simulink model "pacemaker_project_hw_system"  (R2021a)
settings: Solver=FixedStepDiscrete  StartTime=0.0  StopTime=50  FixedStep=1e-3  RelTol=1e-3  EnableMultiTasking=on
model workspace (MAT data in the model file):
  DefaultDataStore = 60
undefined symbols (not defined in the file): A3, A4, D0, D1, D10, D11, D12, D13, D2, D3, D4, D5, D6, D7, D8, D9, PTA0, PTA1, PTA2, PTB11, PTB23, PTB9, PTC11, PTC16, PTC17, PTC2, PTC3, PTC4, PTD0, PTD1, PTD2, PTD3
libraries: frdmk64flib x22, etargetslib x8, dspstat3 x1
settings Model: ExtModeTrigDuration=5  Creator=ali2h  LastModifiedBy=Razan
settings OptimizationCC: EnhancedBackFolding=on  PassReuseOutputArgsAs=Individual arguments  ZeroExternalMemoryAtStartup=off  ZeroInternalMemoryAtStartup=off  MaxStackSize=64  OptimizeBlockOrder=speed  DifferentSizesBufferReuse=on  OptimizationCustomize=off  EfficientTunableParamExpr=on
settings DebuggingCC: ParameterTunabilityLossMsg=error
settings HardwareCC: ProdBitPerPointer=32  ProdBitPerSizeT=32  ProdBitPerPtrDiffT=32  ProdLargestAtomicInteger=Long  ProdLargestAtomicFloat=Double  ProdWordSize=32  ProdHWDeviceType=ARM Compatible->ARM Cortex
settings SFSimCC: MATLABDynamicMemAlloc=off
settings RTWCC: SystemTargetFile=ert.tlc  HardwareBoard=NXP FRDM-K64F  TLCOptions="-aInlineSetEventsForThisBaseRateFcn=TLC_FALSE -aSuppressMultiTaskScheduler=TLC_FALSE  -aRateBasedStepFcn=0"  TemplateMakefile=ert_default_tmf  Toolchain=GNU Tools for ARM Embedded Processors
settings CodeAppCC: ForceParamTrailComments=on  IgnoreCustomStorageClasses=off  OperatorAnnotations=on  SimulinkDataObjDesc=on  SFDataObjDesc=on  InsertBlockDesc=on
settings ERTTargetCC: ExtModeTransport=4  ExtModeMexFile=sendToCommService

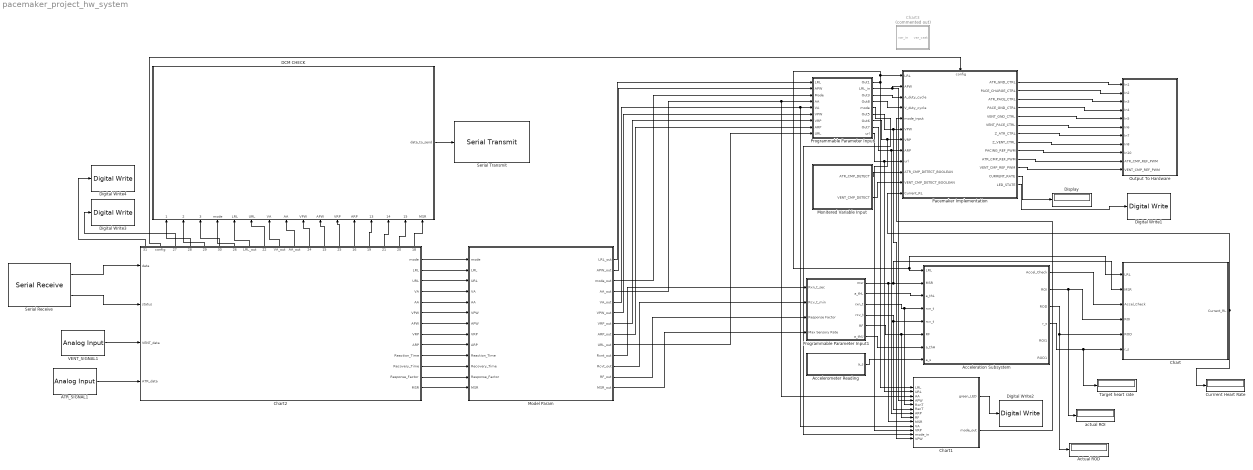
== system pacemaker_project_hw_system ==
  ATR_SIGNAL1 : frdmk64flib/Analog Input  Whichpin=PTB11 (A3)  SampleTime=-1
  Acceleration Subsystem : Subsystem
  Accelerometer Reading : Subsystem
  Actual ROD : Display
  Chart : Stateflow chart  TreatAsAtomicUnit=on
      settings: PortSchema="{\"entries\":[{\"content\":{\"sides\":[{\"content\":{\"connectorIds\":[\"In5\",\"In2\",\"In1\",\"In3\",\"In4\",\"In6\"]},\"type\":\"ConnectorPlacement.EquallySpacedRectSide\",\"uuid\":\"e2faaf11-533e-4519-93e0-9386f0696ab0\"},{\"content\":{\"connectorIds\":[\"Out1\"],\"side\":\"RIGHT\"},\"type\":\"ConnectorPlacement.EquallySpacedRectSide\",\"uuid\":\"3d822896-3a5e-473f-9176-095876908580\"},{\"content\":{\"connectorIds\":[],\"side\":\"TOP\"},\"type\":\"ConnectorPlacement.EquallySpacedRectSide\",\"uuid\":\"9e71e4b9-0a05-47a2-8aca-96ebbea26fb4\"}]},\"type\":\"ConnectorPlacement.EquallySpacedConnector\",\"uuid\":\"95b0b788-f876-4603-914d-e98930842ebd\"}],\"packageUris\":[\"http://schema.mathworks.com/mf0/Connector/R2020b\"],\"version\":\"1.0\"}"
  Chart1 : Stateflow chart  TreatAsAtomicUnit=on
      settings: PortSchema="{\"entries\":[{\"content\":{\"sides\":[{\"content\":{\"connectorIds\":[\"In2\",\"In4\",\"In1\",\"In5\",\"In7\",\"In6\",\"In8\",\"In10\",\"In9\",\"In11\",\"In13\",\"In3\",\"In12\"]},\"type\":\"ConnectorPlacement.EquallySpacedRectSide\",\"uuid\":\"456a7d9e-f2dc-4248-8632-54977d3d0e8d\"},{\"content\":{\"connectorIds\":[\"Out1\",\"Out2\"],\"side\":\"RIGHT\"},\"type\":\"ConnectorPlacement.EquallySpacedRectSide\",\"uuid\":\"93618940-8d2c-4873-bbdd-898375b2771e\"},{\"content\":{\"connectorIds\":[],\"side\":\"TOP\"},\"type\":\"ConnectorPlacement.EquallySpacedRectSide\",\"uuid\":\"193f6807-1d54-4c84-841f-0b1b2c52bae8\"}]},\"type\":\"ConnectorPlacement.EquallySpacedConnector\",\"uuid\":\"4b66c94b-72ab-490e-aaca-3b2f913491ef\"}],\"packageUris\":[\"http://schema.mathworks.com/mf0/Connector/R2020b\"],\"version\":\"1.0\"}"
  Chart2 : Stateflow chart  TreatAsAtomicUnit=on
      settings: PortSchema="{\"entries\":[{\"content\":{\"sides\":[{\"content\":{\"connectorIds\":[\"In1\",\"In2\",\"In3\",\"In4\"]},\"type\":\"ConnectorPlacement.EquallySpacedRectSide\",\"uuid\":\"e0d71676-4635-4cc5-940f-d91659ea50ca\"},{\"content\":{\"connectorIds\":[\"Out2\",\"Out1\",\"Out3\",\"Out4\",\"Out5\",\"Out6\",\"Out7\",\"Out13\",\"Out8\",\"Out9\",\"Out10\",\"Out11\",\"Out12\"],\"side\":\"RIGHT\"},\"type\":\"ConnectorPlacement.EquallySpacedRectSide\",\"uuid\":\"0805dafd-7d20-457a-bd79-7666b5721266\"},{\"content\":{\"connectorIds\":[\"Out31\",\"Out32\",\"Out27\",\"Out28\",\"Out29\",\"Out30\",\"Out26\",\"Out17\",\"Out22\",\"Out23\",\"Out14\",\"Out24\",\"Out15\",\"Out25\",\"Out16\",\"Out19\",\"Out21\",\"Out20\",\"Out18\"],\"side\":\"TOP\"},\"type\":\"ConnectorPlacement.EquallySpacedRectSide\",\"uuid\":\"7dce37fb-9cbe-4aeb-8643-08c0d0009600\"},{\"content\":{\"connectorIds\":[],\"side\":\"BOTTOM\"},\"type\":\"ConnectorPlacement.EquallySpacedRectSide\",\"uuid\":\"8cb6d6e2-e19d-4465-a9e0-7af84bc91401\"}]},\"type\":\"ConnectorPlacement.EquallySpacedConnector\",\"uuid\":\"ce183338-3f92-497d-b3e5-2333b87263be\"}],\"packageUris\":[\"http://schema.mathworks.com/mf0/Connector/R2020b\"],\"version\":\"1.0\"}"
  Chart3 : Stateflow chart  Commented=on  TreatAsAtomicUnit=on
  Currrent Heart Rate : Display
  DCM CHECK : Subsystem
      settings: PortSchema="{\"entries\":[{\"content\":{\"sides\":[{\"content\":{\"connectorIds\":[]},\"type\":\"ConnectorPlacement.EquallySpacedRectSide\",\"uuid\":\"5070fca3-03db-4702-bf74-10cd169506b7\"},{\"content\":{\"connectorIds\":[\"Out1\"],\"side\":\"RIGHT\"},\"type\":\"ConnectorPlacement.EquallySpacedRectSide\",\"uuid\":\"a99172cf-9b5d-4dae-9e4a-5601bc613afa\"},{\"content\":{\"connectorIds\":[],\"side\":\"TOP\"},\"type\":\"ConnectorPlacement.EquallySpacedRectSide\",\"uuid\":\"54f3c445-ca02-417c-9800-ac4eb04fe443\"},{\"content\":{\"connectorIds\":[\"In1\",\"In2\",\"In3\",\"In4\",\"In5\",\"In6\",\"In7\",\"In8\",\"In9\",\"In10\",\"In11\",\"In12\",\"In13\",\"In14\",\"In15\",\"In16\"],\"side\":\"BOTTOM\"},\"type\":\"ConnectorPlacement.EquallySpacedRectSide\",\"uuid\":\"fd0aef12-eb6d-4507-9c8c-5c9fc9d3837d\"}]},\"type\":\"ConnectorPlacement.EquallySpacedConnector\",\"uuid\":\"2a8d6b9e-4cb8-4645-8e28-a1ce966e9c6c\"}],\"packageUris\":[\"http://schema.mathworks.com/mf0/Connector/R2020b\"],\"version\":\"1.0\"}"
  Digital Write1 : frdmk64flib/Digital Write  Whichpin=RED_LED
  Digital Write2 : frdmk64flib/Digital Write  Whichpin=GREEN_LED
  Digital Write3 : frdmk64flib/Digital Write  Whichpin=BLUE_LED
  Digital Write4 : frdmk64flib/Digital Write  Whichpin=PTD1 (D13)
  Display : Display
  Model Param : Subsystem
  Monitered Variable Input : Subsystem
  Output To Hardware : Subsystem
  Pacemaker Implementation : Stateflow chart
      settings: PortSchema="{\"entries\":[{\"content\":{\"sides\":[{\"content\":{\"connectorIds\":[\"In2\",\"In3\",\"In4\",\"In5\",\"In6\",\"In7\",\"In8\",\"In9\",\"In13\",\"In10\",\"In11\",\"In12\"]},\"type\":\"ConnectorPlacement.EquallySpacedRectSide\",\"uuid\":\"2c436aae-0e07-4bda-8b45-2f1ae7c6679d\"},{\"content\":{\"connectorIds\":[\"Out1\",\"Out2\",\"Out3\",\"Out4\",\"Out5\",\"Out6\",\"Out7\",\"Out8\",\"Out9\",\"Out10\",\"Out11\",\"Out12\",\"Out13\"],\"side\":\"RIGHT\"},\"type\":\"ConnectorPlacement.EquallySpacedRectSide\",\"uuid\":\"f66ba986-5db0-4192-b9a8-b5201ea609f2\"},{\"content\":{\"connectorIds\":[\"In1\"],\"side\":\"TOP\"},\"type\":\"ConnectorPlacement.EquallySpacedRectSide\",\"uuid\":\"a7b4d0ec-67b8-4c6f-bf03-752a0cea81dc\"}]},\"type\":\"ConnectorPlacement.EquallySpacedConnector\",\"uuid\":\"6a49745c-0aaa-4843-bb30-dabb7cfb7415\"}],\"packageUris\":[\"http://schema.mathworks.com/mf0/Connector/R2020b\"],\"version\":\"1.0\"}"
  Programmable Parameter Input : Subsystem
  Programmable Parameter Input1 : Subsystem
  Serial Receive : frdmk64flib/Serial Receive  SCIModule=0  Baudrate=uint32(9600)  Parity=None  StopBits=1  HardwareFlowControl=None  ByteOrder=LittleEndian  DataType=uint8  DataLength=29  BlockingMode=off  OutputStatus=on  SampleTime=-1
  Serial Transmit : frdmk64flib/Serial Transmit  SCIModule=0  Baudrate=uint32(9600)  Parity=None  StopBits=1  HardwareFlowControl=None  ByteOrder=LittleEndian  BlockingMode=on  OutputStatus=off
  Target heart rate : Display
  VENT_SIGNAL1 : frdmk64flib/Analog Input  Whichpin=PTC11 (A4)  SampleTime=-1
  actual ROI : Display
  wires:
  Pacemaker Implementation/1(ATR_GND_CTRL) -> Output To Hardware/1(In1)
  Pacemaker Implementation/2(PACE_CHARGE_CTRL) -> Output To Hardware/2(In2)
  Pacemaker Implementation/3(ATR_PACE_CTRL) -> Output To Hardware/3(In3)
  Pacemaker Implementation/4(PACE_GND_CTRL) -> Output To Hardware/4(In4)
  Pacemaker Implementation/5(VENT_GND_CTRL) -> Output To Hardware/5(In5)
  Pacemaker Implementation/6(VENT_PACE_CTRL) -> Output To Hardware/6(In6)
  Pacemaker Implementation/7(Z_ATR_CTRL) -> Output To Hardware/7(In7)
  Pacemaker Implementation/8(Z_VENT_CTRL) -> Output To Hardware/8(In8)
  Pacemaker Implementation/9(PACING_REF_PWM) -> Output To Hardware/9(In10)
  Programmable Parameter Input/2(LRL_in) -> Chart1/5(APW), Pacemaker Implementation/3(APW)
  Programmable Parameter Input/3(Out3) -> Pacemaker Implementation/4(A_duty_cycle)
  Programmable Parameter Input/6(Out5) -> Chart1/12(VPW), Pacemaker Implementation/7(VPW)
  Programmable Parameter Input/7(Out6) -> Chart1/13(VRP), Pacemaker Implementation/8(VRP)
  Programmable Parameter Input/8(Out7) -> Chart1/8(ARP), Pacemaker Implementation/9(ARP)
  Pacemaker Implementation/10(ATR_CMP_REF_PWM) -> Output To Hardware/10(ATR_CMP_REF_PWM)
  Pacemaker Implementation/11(VENT_CMP_REF_PWM) -> Output To Hardware/11(VENT_CMP_REF_PWM)
  Monitered Variable Input/1(ATR_CMP_DETECT) -> Pacemaker Implementation/10(ATR_CMP_DETECT_BOOLEAN)
  Monitered Variable Input/2(VENT_CMP_DETECT) -> Pacemaker Implementation/11(VENT_CMP_DETECT_BOOLEAN)
  Programmable Parameter Input1/2(a_thL) -> Acceleration Subsystem/3(a_thL)
  Programmable Parameter Input1/3(rxn_t) -> Chart1/7(RxnT), Acceleration Subsystem/4(rxn_t)
  Programmable Parameter Input1/4(rcv_t) -> Chart1/6(RecT), Acceleration Subsystem/5(rcv_t)
  Programmable Parameter Input1/5(RF) -> Acceleration Subsystem/6(RF), Chart1/10(RF)
  Programmable Parameter Input1/1(msr) -> Chart1/9(MSR), Acceleration Subsystem/2(MSR), Chart/2(MSR)
  Acceleration Subsystem/1(Accel_Check) -> Chart/1(Accel_Check)
  Acceleration Subsystem/3(ROD) -> Actual ROD/1, Chart/4(ROD)
  Acceleration Subsystem/2(ROI) -> actual ROI/1, Chart/3(ROI)
  Chart/1(Current_RL) -> Currrent Heart Rate/1, Pacemaker Implementation/12(Current_RL)
  Acceleration Subsystem/4(r_s) -> Chart/6(r_s), Target heart rate/1
  Programmable Parameter Input1/6(a_thU) -> Acceleration Subsystem/7(a_thH)
  Pacemaker Implementation/12(CURRENT_RATE) -> Display/1
  Accelerometer Reading/1(a_s) -> Acceleration Subsystem/8(a_s)
  Programmable Parameter Input/4(Out8) -> Pacemaker Implementation/5(V_duty_cycle)
  Model Param/3(mode_out) -> Programmable Parameter Input/3(Mode)
  Model Param/1(LRL_out) -> Programmable Parameter Input/1(LRL)
  Model Param/5(VA_out) -> Chart1/11(VA), Programmable Parameter Input/5(VA)
  Model Param/4(AA_out) -> Chart1/1(AA), Programmable Parameter Input/4(AA)
  Model Param/6(VPW_out) -> Programmable Parameter Input/6(VPW)
  Model Param/2(APW_out) -> Programmable Parameter Input/2(APW)
  Model Param/7(VRP_out) -> Programmable Parameter Input/7(VRP)
  Model Param/8(ARP_out) -> Programmable Parameter Input/8(ARP)
  Model Param/10(Rxnt_out) -> Programmable Parameter Input1/1(Rxn_t_sec)
  Model Param/12(RF_out) -> Programmable Parameter Input1/3(Response Factor)
  Model Param/11(Rcvt_out) -> Programmable Parameter Input1/2(Rcv_t_min)
  Model Param/13(MSR_out) -> Programmable Parameter Input1/4(Max Sensory Rate)
  Programmable Parameter Input/9(url) -> Pacemaker Implementation/13(url), Chart1/4(URL)
  Chart1/1(green_LED) -> Digital Write2/1
  Model Param/9(URL_out) -> Programmable Parameter Input/9(URL)
  Pacemaker Implementation/13(LED_STATE) -> Digital Write1/1
  Programmable Parameter Input/1(Out1) -> Pacemaker Implementation/2(LRL), Chart/5(LRL), Acceleration Subsystem/1(LRL), Chart1/2(LRL)
  Chart2/32(config) -> Pacemaker Implementation/1(config)
  Programmable Parameter Input/5(mode) -> Chart1/3(mode_in)
  Chart1/2(mode_out) -> Pacemaker Implementation/6(mode_input)
  DCM CHECK/1(data_to_send) -> Serial Transmit/1
  ATR_SIGNAL1/1 -> Chart2/4(ATR_data)
  Chart2/28(send_type) -> DCM CHECK/1(send_type)
  VENT_SIGNAL1/1 -> Chart2/3(VENT_data)
  Chart2/29(VENT_egram) -> DCM CHECK/2(VENT_EGRAM)
  Chart2/7(APW) -> Model Param/7(APW)
  Chart2/20(Recovery_Time_out) -> DCM CHECK/15(Recovery_Time)
  Chart2/21(Response_Factor_out) -> DCM CHECK/14(Response_Factor)
  Serial Receive/1 -> Chart2/1(data)
  Serial Receive/2 -> Chart2/2(status)
  Chart2/13(VRP) -> Model Param/8(VRP)
  Chart2/14(AA_out) -> DCM CHECK/8(AA)
  Chart2/12(MSR) -> Model Param/13(MSR)
  Chart2/10(Recovery_Time) -> Model Param/11(Recovery_Time)
  Chart2/9(Reaction_Time) -> Model Param/10(Reaction_Time)
  Chart2/5(AA) -> Model Param/5(AA)
  Chart2/17(LRL_out) -> DCM CHECK/5(LRL)
  Chart2/18(MSR_out) -> DCM CHECK/16(MSR)
  Chart2/25(VRP_out) -> DCM CHECK/11(VRP)
  Chart2/2(mode) -> Model Param/1(mode)
  Chart2/30(ATR_egram) -> DCM CHECK/3(ATR_EGRAM)
  Chart2/8(ARP) -> Model Param/9(ARP)
  Chart2/3(URL) -> Model Param/3(URL)
  Chart2/22(URL_out) -> DCM CHECK/6(URL)
  Chart2/11(Response_Factor) -> Model Param/12(Response_Factor)
  Chart2/1(LRL) -> Model Param/2(LRL)
  Chart2/4(VA) -> Model Param/4(VA)
  Chart2/19(Reaction_Time_out) -> DCM CHECK/13(Reaction_Time)
  Chart2/31(FRNT_END_CTRL) -> Digital Write4/1
  Chart2/23(VA_out) -> DCM CHECK/7(VA)
  Chart2/15(APW_out) -> DCM CHECK/10(APW)
  Chart2/6(VPW) -> Model Param/6(VPW)
  Chart2/24(VPW_out) -> DCM CHECK/9(VPW)
  Chart2/26(mode_out) -> DCM CHECK/4(mode)
  Chart2/16(ARP_out) -> DCM CHECK/12(ARP)
  Chart2/27(blue_LED) -> Digital Write3/1

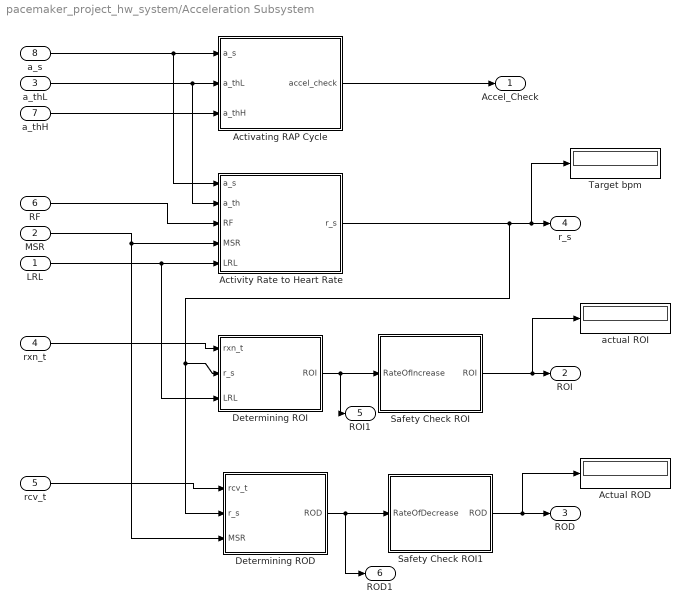
== system pacemaker_project_hw_system/Acceleration Subsystem ==
  LRL : Inport
  MSR : Inport  Port=2
  a_thL : Inport  Port=3
  rxn_t : Inport  Port=4
  rcv_t : Inport  Port=5
  RF : Inport  Port=6
  a_thH : Inport  Port=7
  a_s : Inport  Port=8
  Activating RAP Cycle : MATLAB Function  TreatAsAtomicUnit=on
  Activity Rate to Heart Rate : MATLAB Function  TreatAsAtomicUnit=on
  Actual ROD : Display
  Determining ROD : MATLAB Function  TreatAsAtomicUnit=on
  Determining ROI : MATLAB Function  TreatAsAtomicUnit=on
  Safety Check ROI : MATLAB Function  TreatAsAtomicUnit=on
  Safety Check ROI1 : MATLAB Function  TreatAsAtomicUnit=on
  Target bpm : Display
  actual ROI : Display
  Accel_Check : Outport
  ROI : Outport  Port=2
  ROD : Outport  Port=3
  r_s : Outport  Port=4
  ROI1 : Outport  Port=5
  ROD1 : Outport  Port=6
  wires:
  a_s/1 -> Activating RAP Cycle/1(a_s), Activity Rate to Heart Rate/1(a_s)
  rxn_t/1 -> Determining ROI/1(rxn_t)
  Activating RAP Cycle/1(accel_check) -> Accel_Check/1
  rcv_t/1 -> Determining ROD/1(rcv_t)
  a_thL/1 -> Activating RAP Cycle/2(a_thL), Activity Rate to Heart Rate/2(a_th)
  RF/1 -> Activity Rate to Heart Rate/3(RF)
  MSR/1 -> Activity Rate to Heart Rate/4(MSR), Determining ROD/3(MSR)
  LRL/1 -> Activity Rate to Heart Rate/5(LRL), Determining ROI/3(LRL)
  a_thH/1 -> Activating RAP Cycle/3(a_thH)
  Safety Check ROI/1(ROI) -> actual ROI/1, ROI/1
  Safety Check ROI1/1(ROD) -> Actual ROD/1, ROD/1
  Activity Rate to Heart Rate/1(r_s) -> Target bpm/1, r_s/1, Determining ROD/2(r_s), Determining ROI/2(r_s)
  Determining ROI/1(ROI) -> ROI1/1, Safety Check ROI/1(RateOfIncrease)
  Determining ROD/1(ROD) -> ROD1/1, Safety Check ROI1/1(RateOfDecrease)

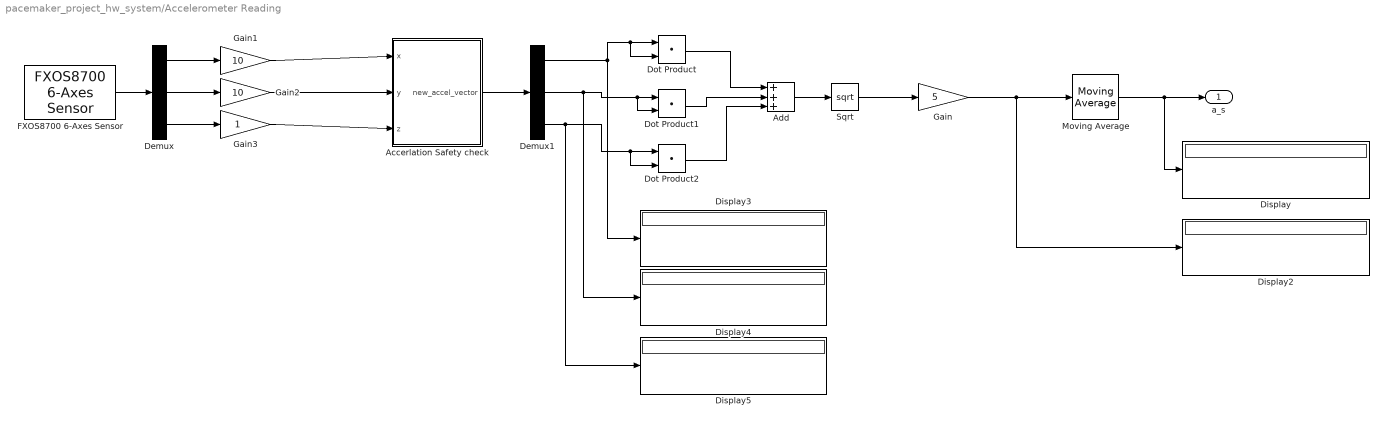
== system pacemaker_project_hw_system/Accelerometer Reading ==
  Accerlation Safety check : MATLAB Function  TreatAsAtomicUnit=on
  Add : Sum  Inputs=+++
  Demux : Demux  Outputs=3
  Demux1 : Demux  Outputs=3
  Display{,2..5} (5 alike) : Display
  Dot Product : DotProduct  InputSameDT=on  OutDataTypeStr=Inherit: Inherit via internal rule
  Dot Product1 : DotProduct  InputSameDT=on  OutDataTypeStr=Inherit: Inherit via internal rule
  Dot Product2 : DotProduct  InputSameDT=on  OutDataTypeStr=Inherit: Inherit via internal rule
  FXOS8700 6-Axes Sensor : frdmk64flib/FXOS8700 6-Axes Sensor  Activesensor=Accelerometer only  ODR=800Hz  HybridODR=400Hz  Accelfullrange=-8g to +8g  SampleTime=-1
  Gain : Gain  Gain=5
  Gain1 : Gain  Gain=10
  Gain2 : Gain  Gain=10
  Gain3 : Gain
  Moving Average : dspstat3/Moving Average  Method=Sliding window  ForgettingFactorPort=off  SpecifyWindowLength=on  WindowLength=15  ForgettingFactor=0.9  SimulateUsing=Code generation
  Sqrt : Sqrt  SaturateOnIntegerOverflow=on
  a_s : Outport
  wires:
  Demux/3 -> Gain3/1
  Sqrt/1 -> Gain/1
  Gain1/1 -> Accerlation Safety check/1(x)
  Add/1 -> Sqrt/1
  Dot Product1/1 -> Add/2
  Demux1/2 -> Display4/1, Dot Product1/2, Dot Product1/1
  Accerlation Safety check/1(new_accel_vector) -> Demux1/1
  Moving Average/1 -> a_s/1, Display/1
  Demux/1 -> Gain1/1
  FXOS8700 6-Axes Sensor/1 -> Demux/1
  Dot Product/1 -> Add/1
  Demux1/1 -> Display3/1, Dot Product/2, Dot Product/1
  Gain/1 -> Display2/1, Moving Average/1
  Demux1/3 -> Display5/1, Dot Product2/2, Dot Product2/1
  Dot Product2/1 -> Add/3
  Demux/2 -> Gain2/1
  Gain3/1 -> Accerlation Safety check/3(z)
  Gain2/1 -> Accerlation Safety check/2(y)

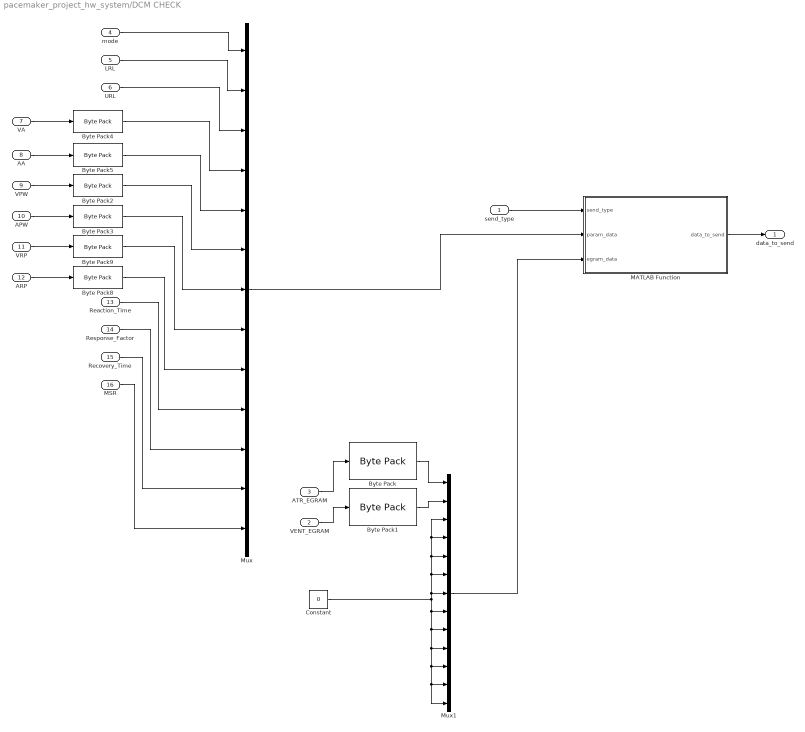
== system pacemaker_project_hw_system/DCM CHECK ==
  send_type : Inport
  VENT_EGRAM : Inport  Port=2  OutDataTypeStr=double
  ATR_EGRAM : Inport  Port=3  OutDataTypeStr=double
  mode : Inport  Port=4  OutDataTypeStr=uint8
  LRL : Inport  Port=5  OutDataTypeStr=uint8
  URL : Inport  Port=6  OutDataTypeStr=uint8
  VA : Inport  Port=7  OutDataTypeStr=single
  AA : Inport  Port=8  OutDataTypeStr=single
  VPW : Inport  Port=9  OutDataTypeStr=single
  APW : Inport  Port=10  OutDataTypeStr=single
  VRP : Inport  Port=11  OutDataTypeStr=uint16
  ARP : Inport  Port=12  OutDataTypeStr=uint16
  Reaction_Time : Inport  Port=13  OutDataTypeStr=uint8
  Response_Factor : Inport  Port=14  OutDataTypeStr=uint8
  Recovery_Time : Inport  Port=15  OutDataTypeStr=uint8
  MSR : Inport  Port=16  OutDataTypeStr=uint8
  Byte Pack : etargetslib/Byte Pack  datatypes={'double'}  byteAlign=1
  Byte Pack1 : etargetslib/Byte Pack  datatypes={'double'}  byteAlign=1
  Byte Pack{2..5} (4 alike) : etargetslib/Byte Pack  datatypes={'single'}  byteAlign=1
  Byte Pack8 : etargetslib/Byte Pack  datatypes={'uint16'}  byteAlign=1
  Byte Pack9 : etargetslib/Byte Pack  datatypes={'uint16'}  byteAlign=1
  Constant : Constant  Value=0  OutDataTypeStr=uint8
  MATLAB Function : MATLAB Function  TreatAsAtomicUnit=on
  Mux : Mux  Inputs=13
  Mux1 : Mux  Inputs=13
  data_to_send : Outport
  wires:
  AA/1 -> Byte Pack5/1
  VA/1 -> Byte Pack4/1
  ARP/1 -> Byte Pack8/1
  LRL/1 -> Mux/2
  VPW/1 -> Byte Pack2/1
  APW/1 -> Byte Pack3/1
  VRP/1 -> Byte Pack9/1
  Byte Pack2/1 -> Mux/6
  Response_Factor/1 -> Mux/11
  mode/1 -> Mux/1
  URL/1 -> Mux/3
  Byte Pack4/1 -> Mux/4
  Byte Pack5/1 -> Mux/5
  Byte Pack3/1 -> Mux/7
  Byte Pack9/1 -> Mux/8
  Byte Pack8/1 -> Mux/9
  Reaction_Time/1 -> Mux/10
  Recovery_Time/1 -> Mux/12
  MSR/1 -> Mux/13
  Constant/1 -> Mux1/11, Mux1/13, Mux1/12, Mux1/10, Mux1/9, Mux1/8, Mux1/4, Mux1/3, Mux1/5, Mux1/6, Mux1/7
  VENT_EGRAM/1 -> Byte Pack1/1
  Byte Pack/1 -> Mux1/1
  ATR_EGRAM/1 -> Byte Pack/1
  Byte Pack1/1 -> Mux1/2
  MATLAB Function/1(data_to_send) -> data_to_send/1
  send_type/1 -> MATLAB Function/1(send_type)
  Mux/1 -> MATLAB Function/2(param_data)
  Mux1/1 -> MATLAB Function/3(egram_data)

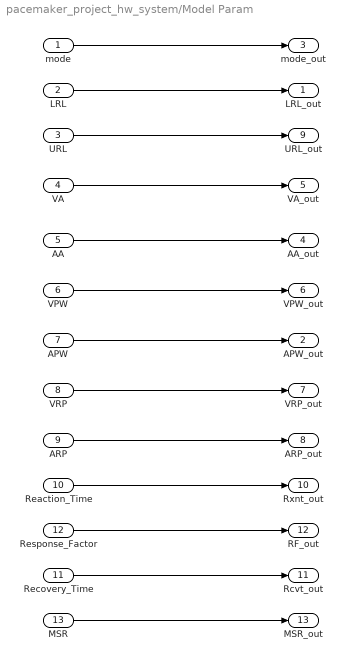
== system pacemaker_project_hw_system/Model Param ==
  mode : Inport
  LRL : Inport  Port=2
  URL : Inport  Port=3
  VA : Inport  Port=4
  AA : Inport  Port=5
  VPW : Inport  Port=6
  APW : Inport  Port=7
  VRP : Inport  Port=8
  ARP : Inport  Port=9
  Reaction_Time : Inport  Port=10
  Recovery_Time : Inport  Port=11
  Response_Factor : Inport  Port=12
  MSR : Inport  Port=13
  LRL_out : Outport
  APW_out : Outport  Port=2
  mode_out : Outport  Port=3
  AA_out : Outport  Port=4
  VA_out : Outport  Port=5
  VPW_out : Outport  Port=6
  VRP_out : Outport  Port=7
  ARP_out : Outport  Port=8
  URL_out : Outport  Port=9
  Rxnt_out : Outport  Port=10
  Rcvt_out : Outport  Port=11
  RF_out : Outport  Port=12
  MSR_out : Outport  Port=13
  wires:
  mode/1 -> mode_out/1
  LRL/1 -> LRL_out/1
  URL/1 -> URL_out/1
  VA/1 -> VA_out/1
  AA/1 -> AA_out/1
  VPW/1 -> VPW_out/1
  APW/1 -> APW_out/1
  VRP/1 -> VRP_out/1
  ARP/1 -> ARP_out/1
  Reaction_Time/1 -> Rxnt_out/1
  Response_Factor/1 -> RF_out/1
  Recovery_Time/1 -> Rcvt_out/1
  MSR/1 -> MSR_out/1

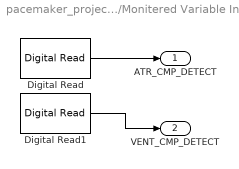
== system pacemaker_project_hw_system/Monitered Variable Input ==
  Digital Read : frdmk64flib/Digital Read  Whichpin=PTC16 (D0)  SampleTime=-1
  Digital Read1 : frdmk64flib/Digital Read  Whichpin=PTC17 (D1)  SampleTime=-1
  ATR_CMP_DETECT : Outport  OutDataTypeStr=boolean
  VENT_CMP_DETECT : Outport  Port=2  OutDataTypeStr=boolean
  wires:
  Digital Read1/1 -> VENT_CMP_DETECT/1
  Digital Read/1 -> ATR_CMP_DETECT/1

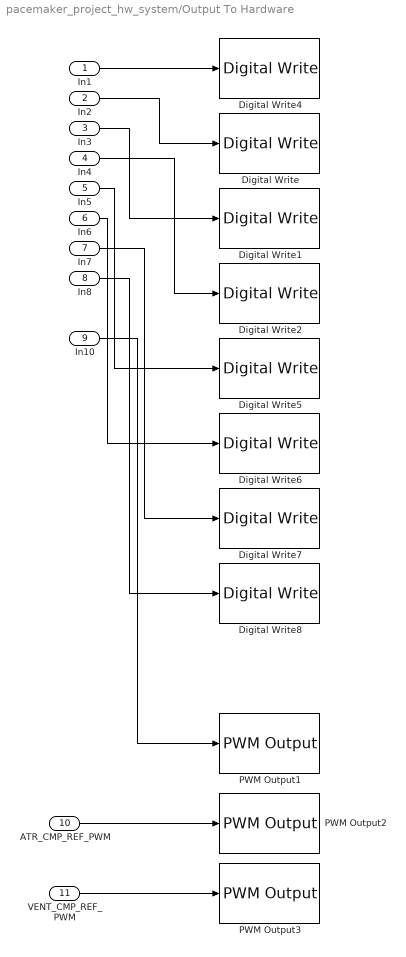
== system pacemaker_project_hw_system/Output To Hardware ==
  In1 : Inport
  In2 : Inport  Port=2
  In3 : Inport  Port=3
  In4 : Inport  Port=4
  In5 : Inport  Port=5
  In6 : Inport  Port=6
  In7 : Inport  Port=7
  In8 : Inport  Port=8
  In10 : Inport  Port=9
  ATR_CMP_REF_PWM : Inport  Port=10
  VENT_CMP_REF_PWM : Inport  Port=11
  Digital Write : frdmk64flib/Digital Write  Whichpin=PTB9 (D2)
  Digital Write1 : frdmk64flib/Digital Write  Whichpin=PTA0 (D8)
  Digital Write2 : frdmk64flib/Digital Write  Whichpin=PTD0 (D10)
  Digital Write4 : frdmk64flib/Digital Write  Whichpin=PTD2 (D11)
  Digital Write5 : frdmk64flib/Digital Write  Whichpin=PTD3 (D12)
  Digital Write6 : frdmk64flib/Digital Write  Whichpin=PTC4 (D9)
  Digital Write7 : frdmk64flib/Digital Write  Whichpin=PTB23 (D4)
  Digital Write8 : frdmk64flib/Digital Write  Whichpin=PTC3 (D7)
  PWM Output1 : frdmk64flib/PWM Output  Whichpin=PTA2 (D5)  InitialFrequency=2000  InitialDutyCycle=0
  PWM Output2 : frdmk64flib/PWM Output  Whichpin=PTC2 (D6)  InitialFrequency=2000  InitialDutyCycle=0
  PWM Output3 : frdmk64flib/PWM Output  Whichpin=PTA1 (D3)  InitialFrequency=2000  InitialDutyCycle=0
  wires:
  In6/1 -> Digital Write6/1
  In7/1 -> Digital Write7/1
  In4/1 -> Digital Write2/1
  In8/1 -> Digital Write8/1
  In3/1 -> Digital Write1/1
  In5/1 -> Digital Write5/1
  In10/1 -> PWM Output1/1
  In1/1 -> Digital Write4/1
  In2/1 -> Digital Write/1
  ATR_CMP_REF_PWM/1 -> PWM Output2/1
  VENT_CMP_REF_PWM/1 -> PWM Output3/1

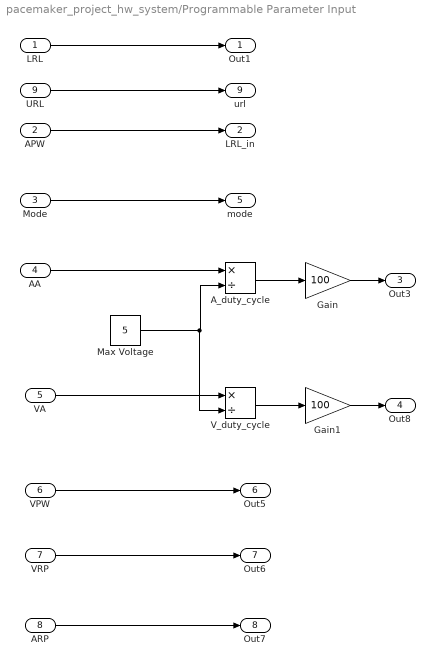
== system pacemaker_project_hw_system/Programmable Parameter Input ==
  LRL : Inport  OutDataTypeStr=uint8
  APW : Inport  Port=2  OutDataTypeStr=single
  Mode : Inport  Port=3  OutDataTypeStr=uint8
  AA : Inport  Port=4  OutDataTypeStr=single
  VA : Inport  Port=5  OutDataTypeStr=single
  VPW : Inport  Port=6  OutDataTypeStr=single
  VRP : Inport  Port=7  OutDataTypeStr=uint16
  ARP : Inport  Port=8  OutDataTypeStr=uint16
  URL : Inport  Port=9  OutDataTypeStr=uint8
  A_duty_cycle : Product  Inputs=*/
  Gain : Gain  Gain=100
  Gain1 : Gain  Gain=100
  Max Voltage : Constant  Value=5  OutDataTypeStr=double
  V_duty_cycle : Product  Inputs=*/
  Out1 : Outport
  LRL_in : Outport  Port=2
  Out3 : Outport  Port=3
  Out8 : Outport  Port=4
  mode : Outport  Port=5  OutDataTypeStr=uint8
  Out5 : Outport  Port=6
  Out6 : Outport  Port=7
  Out7 : Outport  Port=8
  url : Outport  Port=9
  wires:
  Max Voltage/1 -> V_duty_cycle/2, A_duty_cycle/2
  A_duty_cycle/1 -> Gain/1
  APW/1 -> LRL_in/1
  AA/1 -> A_duty_cycle/1
  LRL/1 -> Out1/1
  VPW/1 -> Out5/1
  VRP/1 -> Out6/1
  ARP/1 -> Out7/1
  Mode/1 -> mode/1
  Gain/1 -> Out3/1
  Gain1/1 -> Out8/1
  VA/1 -> V_duty_cycle/1
  V_duty_cycle/1 -> Gain1/1
  URL/1 -> url/1

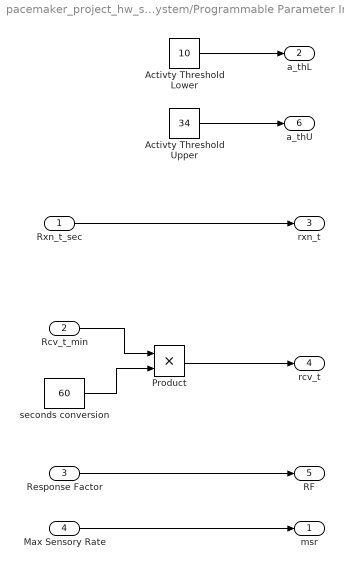
== system pacemaker_project_hw_system/Programmable Parameter Input1 ==
  Rxn_t_sec : Inport
  Rcv_t_min : Inport  Port=2
  Response Factor : Inport  Port=3
  Max Sensory Rate : Inport  Port=4
  Activty Threshold Lower : Constant  Value=10  OutDataTypeStr=double
  Activty Threshold Upper : Constant  Value=34  OutDataTypeStr=double
  Product : Product
  "seconds conversion " : Constant  Value=60  OutDataTypeStr=double
  msr : Outport
  a_thL : Outport  Port=2
  rxn_t : Outport  Port=3
  rcv_t : Outport  Port=4
  RF : Outport  Port=5
  a_thU : Outport  Port=6
  wires:
  Activty Threshold Lower/1 -> a_thL/1
  Response Factor/1 -> RF/1
  Rcv_t_min/1 -> Product/1
  "seconds conversion "/1 -> Product/2
  Activty Threshold Upper/1 -> a_thU/1
  Rxn_t_sec/1 -> rxn_t/1
  Product/1 -> rcv_t/1
  Max Sensory Rate/1 -> msr/1

== matlab function pacemaker_project_hw_system/Acceleration Subsystem/Determining ROI ==
  data: rxn_t input; ROI output; r_s input; LRL input
function ROI = fcn(rxn_t, r_s, LRL)

ROI = (r_s-LRL)/(rxn_t)
end

== matlab function pacemaker_project_hw_system/Acceleration Subsystem/Activity Rate to Heart Rate ==
  data: a_s input; a_th input; r_s output; RF input; MSR input; LRL input
function r_s = fcn(a_s, a_th, RF, MSR, LRL)

factor = RF*(34-10)/16;
slope = (MSR-LRL)/(35-10-factor);
y = slope*(a_s-a_th) + LRL;
    if MSR == LRL
        r_s = (LRL+MSR)/2;
    else
        if y<=LRL
            r_s= LRL;
        elseif MSR<=y
            r_s= MSR;
        else
            r_s =y;
        end
    end
    
%         %r_s = ((bool)*LRL +((LRL<y)&(y<MSR))*y + (MSR<=y)*MSR)/2;
%     else
%         r_s = (y<=LRL)*LRL +((LRL<y)&(y<MSR))*y + (MSR<=y)*MSR;
%     end 
end

== stateflow chart pacemaker_project_hw_system/Pacemaker Implementation ==
  state Initialization_Mode
    entry:
    %Initial State before mode begins pacing
    if mode_input == 2
    LED_STATE = true;
    end
    mode = mode_input;
    configured = false;
  state AOOR_Initial
    %CHARGE_C22
    entry:
    ATR_PACE_CTRL = false;
    VENT_PACE_CTRL = false;
    PACING_REF_PWM = A_duty_cycle;
    PACE_CHARGE_CTRL = true;
    %DISCHARGE_C21
    PACE_GND_CTRL = true;
    VENT_PACE_CTRL = false;
    Z_ATR_CTRL = false;
    Z_VENT_CTRL = false;
    ATR_PACE_CTRL = false;
    ATR_GND_CTRL = true;
    VENT_GND_CTRL = false;
    LED_STATE = false;
    configured= config;
  state AOO_Initial
    %CHARGE_C22
    entry:
    ATR_PACE_CTRL = false;
    VENT_PACE_CTRL = false;
    PACING_REF_PWM = A_duty_cycle;
    PACE_CHARGE_CTRL = true;
    %DISCHARGE_C21
    PACE_GND_CTRL = true;
    VENT_PACE_CTRL = false;
    Z_ATR_CTRL = false;
    Z_VENT_CTRL = false;
    ATR_PACE_CTRL = false;
    ATR_GND_CTRL = true;
    VENT_GND_CTRL = false;
    LED_STATE = false;
    configured= config;
  state AOO_Pacing
    %DISCHARGE_C22_and_CHARGE_C21
    entry:
    PACE_CHARGE_CTRL = false;
    PACE_GND_CTRL = true;
    ATR_PACE_CTRL = true;
    ATR_GND_CTRL = false;
    Z_ATR_CTRL = false;
    Z_VENT_CTRL = false;
    VENT_GND_CTRL = false;
    VENT_PACE_CTRL = false;
    LED_STATE = false
  state AOOR_Pacing
    %DISCHARGE_C22_and_CHARGE_C21
    entry:
    PACE_CHARGE_CTRL = false;
    PACE_GND_CTRL = true;
    ATR_PACE_CTRL = true;
    ATR_GND_CTRL = false;
    Z_ATR_CTRL = false;
    Z_VENT_CTRL = false;
    VENT_GND_CTRL = false;
    VENT_PACE_CTRL = false;
    LED_STATE = true;
  state VOO_Initial
    %CHARGE_C22
    entry:
    ATR_PACE_CTRL = false;
    VENT_PACE_CTRL = false;
    PACING_REF_PWM = V_duty_cycle;
    PACE_CHARGE_CTRL = true;
    %DISCHARGE_C21
    PACE_GND_CTRL = true;
    VENT_PACE_CTRL = false;
    Z_ATR_CTRL = false;
    Z_VENT_CTRL = false;
    ATR_PACE_CTRL = false;
    ATR_GND_CTRL = false;
    VENT_GND_CTRL = true;
    LED_STATE = true;
    configured= config;
  state VOO_Pacing
    %DISCHARGE_C22_and_CHARGE_C21
    entry:
    PACE_CHARGE_CTRL = false;
    PACE_GND_CTRL = true;
    ATR_PACE_CTRL = false;
    ATR_GND_CTRL = false;
    Z_ATR_CTRL = false;
    Z_VENT_CTRL = false;
    VENT_GND_CTRL = false;
    VENT_PACE_CTRL = true;
    LED_STATE = false;
  state VOOR_Initial
    %CHARGE_C22
    entry:
    ATR_PACE_CTRL = false;
    VENT_PACE_CTRL = false;
    PACING_REF_PWM = V_duty_cycle;
    PACE_CHARGE_CTRL = true;
    %DISCHARGE_C21
    PACE_GND_CTRL = true;
    VENT_PACE_CTRL = false;
    Z_ATR_CTRL = false;
    Z_VENT_CTRL = false;
    ATR_PACE_CTRL = false;
    ATR_GND_CTRL = false;
    VENT_GND_CTRL = true;
    LED_STATE = false;
    configured= config;
  state VOOR_Pacing
    %DISCHARGE_C22_and_CHARGE_C21
    entry:
    PACE_CHARGE_CTRL = false;
    PACE_GND_CTRL = true;
    ATR_PACE_CTRL = false;
    ATR_GND_CTRL = false;
    Z_ATR_CTRL = false;
    Z_VENT_CTRL = false;
    VENT_GND_CTRL = false;
    VENT_PACE_CTRL = true;
    LED_STATE = true;
    CURRENT_RATE = Current_RL;
  state AAI_Initial1
    %CHARGE_C22
    entry:
    ATR_PACE_CTRL = false;
    VENT_PACE_CTRL = false;
    PACING_REF_PWM = A_duty_cycle;
    PACE_CHARGE_CTRL = true;
    %DISCHARGE_C21
    PACE_GND_CTRL = true;
    VENT_PACE_CTRL = false;
    Z_ATR_CTRL = false;
    Z_VENT_CTRL = false;
    ATR_PACE_CTRL = false;
    ATR_GND_CTRL = true;
    VENT_GND_CTRL = false;
    LED_STATE = false;
    %Sensing
    %FRONTEND_CTRL = true;
    ATR_CMP_REF_PWM = (3.5/5*100);
    LED_STATE_BLUE = false;
    configured= config;
  state AAI_Pacing1
    %DISCHARGE_C22_and_CHARGE_C21
    entry:
    PACE_CHARGE_CTRL = false;
    PACE_GND_CTRL = true;
    ATR_PACE_CTRL = true;
    ATR_GND_CTRL = false;
    Z_ATR_CTRL = false;
    Z_VENT_CTRL = false;
    VENT_GND_CTRL = false;
    VENT_PACE_CTRL = false;
    LED_STATE_BLUE = true;
  state AAIR_Initial
    %CHARGE_C22
    entry:
    ATR_PACE_CTRL = false;
    VENT_PACE_CTRL = false;
    PACING_REF_PWM = A_duty_cycle;
    PACE_CHARGE_CTRL = true;
    %DISCHARGE_C21
    PACE_GND_CTRL = true;
    VENT_PACE_CTRL = false;
    Z_ATR_CTRL = false;
    Z_VENT_CTRL = false;
    ATR_PACE_CTRL = false;
    ATR_GND_CTRL = true;
    VENT_GND_CTRL = false;
    LED_STATE = false;
    %Sensing
    %FRONTEND_CTRL = true;
    ATR_CMP_REF_PWM = (3.5/5*100);
    LED_STATE_BLUE = false;
    configured= config;
  state AAIR_Pacing
    %DISCHARGE_C22_and_CHARGE_C21
    entry:
    PACE_CHARGE_CTRL = false;
    PACE_GND_CTRL = true;
    ATR_PACE_CTRL = true;
    ATR_GND_CTRL = false;
    Z_ATR_CTRL = false;
    Z_VENT_CTRL = false;
    VENT_GND_CTRL = false;
    VENT_PACE_CTRL = false;
    LED_STATE_BLUE = true;
  state AAI_Proxy
    %DISCHARGE_C21
    entry:
    PACE_GND_CTRL = true;
    VENT_PACE_CTRL = false;
    Z_ATR_CTRL = false;
    Z_VENT_CTRL = false;
    ATR_PACE_CTRL = false;
    ATR_GND_CTRL = true;
    VENT_GND_CTRL = false;
    LED_STATE = true;
    %CHARGE_C22
    ATR_PACE_CTRL = false;
    VENT_PACE_CTRL = false;
    PACING_REF_PWM = A_duty_cycle;
    PACE_CHARGE_CTRL = true;
    LED_STATE_BLUE = false;
  state AAIR_Proxy
    %DISCHARGE_C21
    entry:
    PACE_GND_CTRL = true;
    VENT_PACE_CTRL = false;
    Z_ATR_CTRL = false;
    Z_VENT_CTRL = false;
    ATR_PACE_CTRL = false;
    ATR_GND_CTRL = true;
    VENT_GND_CTRL = false;
    LED_STATE = true;
    %CHARGE_C22
    ATR_PACE_CTRL = false;
    VENT_PACE_CTRL = false;
    PACING_REF_PWM = A_duty_cycle;
    PACE_CHARGE_CTRL = true;
    LED_STATE_BLUE = false;
  state VVIR_Initial
    %CHARGE_C22
    entry:
    VENT_PACE_CTRL = false;
    PACING_REF_PWM = V_duty_cycle;
    PACE_CHARGE_CTRL = true;
    ATR_PACE_CTRL = false;
    %DISCHARGE_C21
    PACE_GND_CTRL = true;
    VENT_PACE_CTRL = false;
    Z_ATR_CTRL = false;
    Z_VENT_CTRL = false;
    ATR_PACE_CTRL = false;
    ATR_GND_CTRL = false;
    VENT_GND_CTRL = true;
    LED_STATE = false;
    LED_STATE_BLUE = false;
    %sensing
    %FRONTEND_CTRL = true;
    VENT_CMP_REF_PWM = (3.5/5*100);
    configured= config;
  state VVIR_Pacing
    %DISCHARGE_C22_and_CHARGE_C21
    entry:
    PACE_CHARGE_CTRL = false;
    PACE_GND_CTRL = true;
    ATR_PACE_CTRL = false;
    ATR_GND_CTRL = false;
    Z_ATR_CTRL = false;
    Z_VENT_CTRL = false;
    VENT_GND_CTRL = false;
    VENT_PACE_CTRL = true;
    LED_STATE_BLUE = true
  state VVI_Initial1
    %CHARGE_C22
    entry:
    VENT_PACE_CTRL = false;
    PACING_REF_PWM = V_duty_cycle;
    PACE_CHARGE_CTRL = true;
    ATR_PACE_CTRL = false;
    %DISCHARGE_C21
    PACE_GND_CTRL = true;
    VENT_PACE_CTRL = false;
    Z_ATR_CTRL = false;
    Z_VENT_CTRL = false;
    ATR_PACE_CTRL = false;
    ATR_GND_CTRL = false;
    VENT_GND_CTRL = true;
    LED_STATE = false;
    LED_STATE_BLUE = false;
    %sensing
    %FRONTEND_CTRL = true;
    VENT_CMP_REF_PWM = (3.5/5*100);
    configured= config;
  state VVI_Pacing1
    %DISCHARGE_C22_and_CHARGE_C21
    entry:
    PACE_CHARGE_CTRL = false;
    PACE_GND_CTRL = true;
    ATR_PACE_CTRL = false;
    ATR_GND_CTRL = false;
    Z_ATR_CTRL = false;
    Z_VENT_CTRL = false;
    VENT_GND_CTRL = false;
    VENT_PACE_CTRL = true;
    LED_STATE_BLUE = true
  state VVIR_Proxy
    %DISCHARGE_C21
    entry:
    PACE_GND_CTRL = true;
    VENT_PACE_CTRL = false;
    Z_ATR_CTRL = false;
    Z_VENT_CTRL = false;
    ATR_PACE_CTRL = false;
    ATR_GND_CTRL = false;
    VENT_GND_CTRL = true;
    LED_STATE = true;
    %CHARGE_C22
    ATR_PACE_CTRL = false;
    VENT_PACE_CTRL = false;
    PACING_REF_PWM = V_duty_cycle;
    PACE_CHARGE_CTRL = true;
  state VVI_Proxy
    %DISCHARGE_C21
    entry:
    PACE_GND_CTRL = true;
    VENT_PACE_CTRL = false;
    Z_ATR_CTRL = false;
    Z_VENT_CTRL = false;
    ATR_PACE_CTRL = false;
    ATR_GND_CTRL = false;
    VENT_GND_CTRL = true;
    LED_STATE = true;
    %CHARGE_C22
    ATR_PACE_CTRL = false;
    VENT_PACE_CTRL = false;
    PACING_REF_PWM = V_duty_cycle;
    PACE_CHARGE_CTRL = true;
  AAIR_Initial -> Initialization_Mode [order 3] : [config]
  VOOR_Initial -> Initialization_Mode [order 2] : [config]
  VVIR_Initial -> Initialization_Mode [order 3] : [config]
  Initialization_Mode -> AOOR_Initial [order 5] : [mode == 5]
  (default) -> Initialization_Mode
  Initialization_Mode -> VOOR_Initial [order 6] : [mode == 6]
  Initialization_Mode -> AAIR_Initial [order 7] : [mode == 7]
  Initialization_Mode -> VVI_Initial1 [order 4] : [mode == 4]
  Initialization_Mode -> AAI_Initial1 [order 3] : [mode == 3]
  Initialization_Mode -> VOO_Initial [order 2] : [mode == 2]
  Initialization_Mode -> VVIR_Initial [order 8] : [mode == 8]
  AOO_Initial -> Initialization_Mode [order 2] : [config]
  Initialization_Mode -> AOO_Initial [order 1] : [mode== 1]
  VOO_Initial -> Initialization_Mode [order 2] : [config]
  AAI_Initial1 -> Initialization_Mode [order 3] : [config]
  AOOR_Initial -> Initialization_Mode [order 2] : [config]
  VVI_Initial1 -> Initialization_Mode [order 3] : [config]
  AOO_Initial -> AOO_Pacing [order 1] : after((30000/cast(LRL, 'single')-APW), msec)
  AOOR_Initial -> AOOR_Pacing [order 1] : after((30000/cast(Current_RL, 'single')-APW), msec)
  AOO_Pacing -> AOO_Initial : after(APW, msec)
  AOOR_Pacing -> AOOR_Initial : after(APW, msec)
  VOO_Initial -> VOO_Pacing [order 1] : after((30000/cast(LRL, 'single')-VPW), msec)
  VOOR_Initial -> VOOR_Pacing [order 1] : after((30000/cast(Current_RL, 'single')-VPW), msec)
  VOO_Pacing -> VOO_Initial : after(VPW, msec)
  VOOR_Pacing -> VOOR_Initial : after(VPW, msec)
  AAI_Initial1 -> AAI_Pacing1 [order 2] : after(30000/cast(LRL,'single') - APW - cast(ARP,'single'), msec)
  AAIR_Initial -> AAIR_Pacing [order 2] : after(30000/cast(Current_RL, 'single') - APW - cast(ARP, 'single'), msec)
  AAI_Pacing1 -> AAI_Proxy : after(APW, msec)
  AAIR_Pacing -> AAIR_Proxy : after(APW, msec)
  AAI_Proxy -> AAI_Initial1 : after(ARP, msec)
  AAI_Initial1 -> AAI_Proxy [order 1] : [ATR_CMP_DETECT_BOOLEAN == true]
  AAIR_Proxy -> AAIR_Initial : after(ARP, msec)
  AAIR_Initial -> AAIR_Proxy [order 1] : [ATR_CMP_DETECT_BOOLEAN == true]
  VVIR_Initial -> VVIR_Pacing [order 2] : after(30000/cast(Current_RL, 'single') - cast(VRP, 'single')-VPW, msec)
  VVI_Initial1 -> VVI_Pacing1 [order 2] : after(30000/cast(LRL, 'single') - cast(VRP,'single')-VPW, msec)
  VVIR_Pacing -> VVIR_Proxy : after(VPW, msec)
  VVI_Pacing1 -> VVI_Proxy : after(VPW, msec)
  VVIR_Proxy -> VVIR_Initial : after(VRP, msec)
  VVIR_Initial -> VVIR_Proxy [order 1] : [VENT_CMP_DETECT_BOOLEAN == true]
  VVI_Proxy -> VVI_Initial1 : after(VRP, msec)
  VVI_Initial1 -> VVI_Proxy [order 1] : [VENT_CMP_DETECT_BOOLEAN == true]
  data: config input; LRL input; APW input; ATR_GND_CTRL output; PACE_CHARGE_CTRL output; ATR_PACE_CTRL output; PACE_GND_CTRL output; VENT_GND_CTRL output; VENT_PACE_CTRL output; Z_ATR_CTRL output; Z_VENT_CTRL output; A_duty_cycle input double; V_duty_cycle input; PACING_REF_PWM output; mode_input input double; VPW input; VRP input; ARP input; ATR_CMP_REF_PWM output; VENT_CMP_REF_PWM output; ATR_CMP_DETECT_BOOLEAN input boolean; VENT_CMP_DETECT_BOOLEAN input boolean; Current_RL input; CURRENT_RATE output; URL_contigency local; url input; LED_STATE_BLUE local; LRL_float local; Current_RL_float local; ARP_float local; LED_STATE output; mode local double; configured local

== matlab function pacemaker_project_hw_system/Acceleration Subsystem/Determining ROD ==
  data: rcv_t input; ROD output; r_s input; MSR input
function ROD = fcn(rcv_t, r_s, MSR)

ROD = (MSR-r_s)/(rcv_t)
end

== matlab function pacemaker_project_hw_system/Acceleration Subsystem/Activating RAP Cycle ==
  data: a_s input; a_thL input; accel_check output; a_thH input
function accel_check = fcn(a_s, a_thL, a_thH)
if a_s<a_thL
    accel_check = 0;
elseif a_s>a_thH
    accel_check = 2;
else
    accel_check = 1;
end

== stateflow chart pacemaker_project_hw_system/Chart ==
  state Initialization_State
    entry:
    Current_RL = LRL;
    TRL = r_s;
    Rate_of_Increase = ROI;
    Rate_of_Decrease = ROD;
  state Looping_State
    entry:
    Current_RL = Current_RL;
    TRL = r_s;
    Rate_of_Increase = ROI;
    Rate_of_Decrease = ROD;
  state Activity_LowOrHigh
    entry:
    if Accel_Check == 0
    TRL = LRL
    elseif Accel_Check == 2
    TRL = MSR
    end
  state Increase_HeartRate
    entry:
    if Current_RL + Rate_of_Increase > MSR
    Current_RL = MSR
    elseif Current_RL + Rate_of_Increase > TRL
    Current_RL = TRL
    else
    Current_RL = Current_RL + Rate_of_Increase
    end
  state Decrease_HeartRate
    entry:
    if Current_RL - Rate_of_Decrease < LRL
    Current_RL = LRL
    elseif Current_RL - Rate_of_Increase < TRL
    Current_RL = TRL
    else
    Current_RL = Current_RL - Rate_of_Decrease
    end
  Looping_State -> Activity_LowOrHigh [order 2] : after(1, sec)
  (default) -> Initialization_State
  Initialization_State -> Activity_LowOrHigh [order 2]
  Initialization_State -> (junction 5) [order 1] : [Accel_Check == 1]
  Looping_State -> (junction 5) [order 1] : after(1, sec)[Accel_Check == 1]
  (junction 38) -> Looping_State
  Activity_LowOrHigh -> (junction 5)
  (junction 5) -> Decrease_HeartRate [order 1] : [Current_RL > TRL]
  (junction 5) -> Increase_HeartRate [order 3] : [Current_RL < TRL]
  (junction 5) -> (junction 38) [order 2] : [Current_RL == TRL]
  Increase_HeartRate -> (junction 38)
  Decrease_HeartRate -> (junction 38)
  data: Accel_Check input; TRL local; MSR input; ROI input; Rate_of_Increase local; ROD input; Rate_of_Decrease local; LRL input; Current_RL output; r_s input

== matlab function pacemaker_project_hw_system/Acceleration Subsystem/Safety Check ROI1 ==
  data: RateOfDecrease input; ROD output
function ROD = fcn(RateOfDecrease)
if RateOfDecrease<0
    ROD = cast(0,'double');
elseif RateOfDecrease>1.2
    ROD = cast(1.2,'double');
else
    ROD = cast(RateOfDecrease,'double');
  
end

== matlab function pacemaker_project_hw_system/Acceleration Subsystem/Safety Check ROI ==
  data: RateOfIncrease input; ROI output
function ROI = fcn(RateOfIncrease)
if RateOfIncrease<0
    ROI = cast(0, 'double');
elseif RateOfIncrease>7
    ROI = cast(7, 'double');
else
    ROI = cast(RateOfIncrease, 'double');
  
end

== stateflow chart pacemaker_project_hw_system/Chart1 ==
  state LED_TEST
    entry:
    LED = false;
    if (mode_in == 1)
    mode_out = 1
    LED = true;
    end
    if (mode_in == 2)
    mode_out = 2
    LED = true;
    end
    if (mode_in == 3)
    mode_out = 3
    LED = true;
    end
    if (mode_in == 4)
    mode_out = 4
    LED = true;
    end
    if (mode_in == 5)
    mode_out = 5
    LED = true;
    end
    if (mode_in == 6)
    mode_out = 6
    LED = true;
    end
    if (mode_in == 7)
    mode_out = 7
    LED = true;
    end
    if (mode_in == 8 )
    mode_out = 8
    LED = true;
    end
    green_LED = false;
    red_LED = false;
  state LED_ON
    entry:
    green_LED = true;
  (default) -> LED_TEST
  LED_TEST -> LED_ON : [LED == true]
  LED_ON -> LED_TEST : after(3, sec)
  data: green_LED output; LED local; AA input; LRL input; mode_in input; URL input; APW input; red_LED local; RecT input; RxnT input; ARP input; MSR input; RF input; VA input; VPW input; VRP input; mode_out output double

== stateflow chart pacemaker_project_hw_system/Chart2 ==
  settings: executeAtInitialization=1
  state SEND_EGRAM
    entry:
    send_type = 1;
    blue_LED = false;
    ATR_egram = ATR_data;
    VENT_egram =VENT_data;
  state CHECKPOINT
    entry:
    index = 3; %Starting index
    %Mode
    mode_check = data(index);
    index = index + 1;
    %Programmable Parameters - for non-rate adaptive modes
    LRL_check = data(index);
    index = index + 1;
    URL_check = data(index);
    index = index + 1;
    VA_check = typecast(data(index:index+3),'single');
    index = index + 4;
    AA_check = typecast(data(index:index+3),'single');
    index = index + 4;
    VPW_check = typecast(data(index:index+3),'single');
    index = index + 4;
    APW_check = typecast(data(index:index+3),'single');
    index = index + 4;
    VRP_check = typecast(data(index:index+1),'uint16');
    index = index + 2;
    ARP_check = typecast(data(index:index+1),'uint16');
    index = index + 2;
    %Rate Adaptive Parameters
    Reaction_Time_check = data(index);
    index = index + 1;
    Response_Factor_check = data(index);
    index = index + 1;
    Recovery_Time_check = data(index);;
    index = index + 1;
    MSR_check = data(index);
    %This state is reached once the check varaibles have been set
    % Its purpose is to set the output variables that are sent back to the DCM to be checked
    %OUTPUTS
    mode_out = mode_check ;%what should be default mode
    LRL_out = LRL_check;
    URL_out = URL_check;
    VA_out = VA_check;
    AA_out = AA_check;
    VPW_out = VPW_check;
    APW_out = APW_check;
    VRP_out = VRP_check;
    ARP_out = ARP_check;
    Reaction_Time_out = Reaction_Time_check;
    Response_Factor_out = Response_Factor_check;
    Recovery_Time_out = Recovery_Time_check;
    MSR_out = MSR_check;
    blue_LED = true;
  state INITIAL
    entry:
    mode = 1 ;%what should be default mode
    LRL = 60;
    URL = 120;
    VA = 3.5;
    AA = 3.5;
    VPW = 0.4;
    APW = 0.4;
    VRP = 320;
    ARP = 500;
    Reaction_Time = 30;
    Response_Factor = 8;
    Recovery_Time = 5;
    MSR = 120;
    FRNT_END_CTRL = true;
  state STANDBY
    %Waiting for COM
    config = false;
  state MODEL_PARAM1
    %this state can only be reached if the GO_AHEAD
    %in the DCM is successful
    entry:
    mode = mode_check ;%what should be default mode
    LRL = LRL_check;
    URL = URL_check;
    VA = VA_check;
    AA = AA_check;
    VPW = VPW_check;
    APW = APW_check;
    VRP = VRP_check;
    ARP = ARP_check;
    Reaction_Time = Reaction_Time_check;
    Response_Factor = Response_Factor_check;
    Recovery_Time = Recovery_Time_check;
    MSR = MSR_check;
    blue_LED = false;
    config = true;
  SEND_EGRAM -> STANDBY
  (junction 17) -> SEND_EGRAM [order 2] : [data(1) == hex2dec('33')]
  CHECKPOINT -> STANDBY
  (default) -> INITIAL
  (junction 17) -> STANDBY [order 3]
  INITIAL -> STANDBY
  STANDBY -> (junction 17) : [status == 0]
  (junction 17) -> (junction 21) [order 1] : [data(1)==hex2dec('16')]
  (junction 21) -> CHECKPOINT [order 1] : [data(2)== hex2dec('55')]
  (junction 21) -> MODEL_PARAM1 [order 2] : [data(2) == hex2dec('22')]
  MODEL_PARAM1 -> STANDBY
  data: data input uint8; status input uint8; LRL output uint8; mode output uint8; URL output uint8; VA output single; AA output single; VPW output single; APW output single; ARP output uint16; Reaction_Time output uint8; Recovery_Time output uint8; Response_Factor output uint8; MSR output uint8; index local; VRP output uint16; AA_check local single; APW_check local single; ARP_check local uint16; LRL_check local uint8; MSR_check local uint8; Reaction_Time_check local uint8; Recovery_Time_check local uint8; Response_Factor_check local uint8; URL_check local uint8; VA_check local single; VPW_check local single; VRP_check local uint16; mode_check local uint8; AA_out output single; APW_out output single; ARP_out output uint16; LRL_out output uint8; MSR_out output uint8; Reaction_Time_out output uint8; Recovery_Time_out output uint8; Response_Factor_out output uint8; URL_out output uint8; VA_out output single; VPW_out output single; VRP_out output uint16; mode_out output uint8; blue_LED output; send_type output; VENT_egram output; ATR_egram output; VENT_data input double; ATR_data input double; FRNT_END_CTRL output; config output

== stateflow chart pacemaker_project_hw_system/Chart3 ==
  state CAST
    entry:
    var_cast = var_in;
  (default) -> CAST
  data: var_cast output; var_in input

== matlab function pacemaker_project_hw_system/Accelerometer Reading/Accerlation Safety check ==
  data: x input; new_accel_vector output; y input; z input
function new_accel_vector = fcn(x,y,z)
% if elevator
if (z >= x*5)&& (z>=y*5)
    new_accel_vector = [0,0,1]; %rest
end
% if car
if (x >= z*5)&& (x>=y*5)
    new_accel_vector = [0,0,1]; %rest
end
new_accel_vector = [x,y,z];
end

== matlab function pacemaker_project_hw_system/DCM CHECK/MATLAB Function ==
  data: send_type input; data_to_send output; param_data input; egram_data input
function data_to_send = fcn(send_type, param_data, egram_data)
if send_type == 0
    data_to_send = param_data;
elseif send_type == 1
    data_to_send = egram_data;
else
    data_to_send = param_data;
end

end
